simulink model "CELL_MODEL"  (R2017a)
settings: Solver=VariableStepAuto  StartTime=0.0  StopTime=82  RelTol=1e-3
undefined symbols (not defined in the file): C1_LUT, Capacity_LUT, cell_area, cell_Cp_heat, cell_mass, Em_LUT, h_conv, R0_LUT, R1_LUT, SOC_LUT, T_init, Temperature_LUT
settings Model: Creator=Win  LastModifiedBy=Win

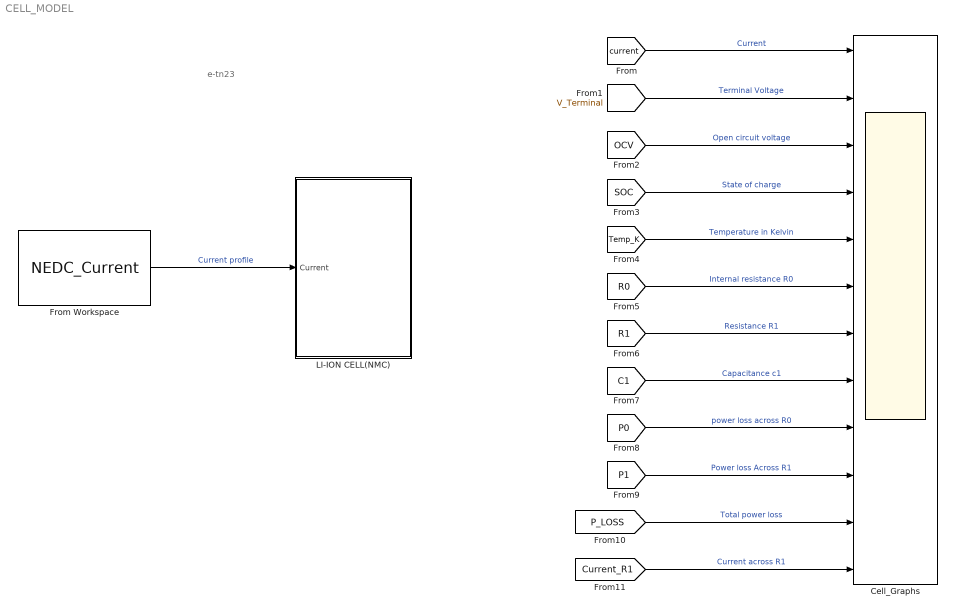
== system CELL_MODEL ==
  note: e-tn23
  Cell_Graphs : Scope  NumInputPorts=12
  From Workspace : FromWorkspace  VariableName=NEDC_Current  SampleTime=0
  LI-ION CELL(NMC) : Subsystem
  wires:
  From Workspace/1 -> LI-ION CELL(NMC)/1(Current)  "Current profile"
  [P_LOSS] -> Cell_Graphs/11  "Total power loss"
  [P1] -> Cell_Graphs/10  "Power loss Across R1"
  [P0] -> Cell_Graphs/9  "power loss across R0"
  [C1] -> Cell_Graphs/8  "Capacitance c1"
  [R1] -> Cell_Graphs/7  "Resistance R1"
  [R0] -> Cell_Graphs/6  "Internal resistance R0"
  [Temp_K] -> Cell_Graphs/5  "Temperature in Kelvin"
  [SOC] -> Cell_Graphs/4  "State of charge"
  [OCV] -> Cell_Graphs/3  "Open circuit voltage"
  [V_Terminal] -> Cell_Graphs/2  "Terminal Voltage"
  [current] -> Cell_Graphs/1  "Current"
  [Current_R1] -> Cell_Graphs/12  "Current across R1"

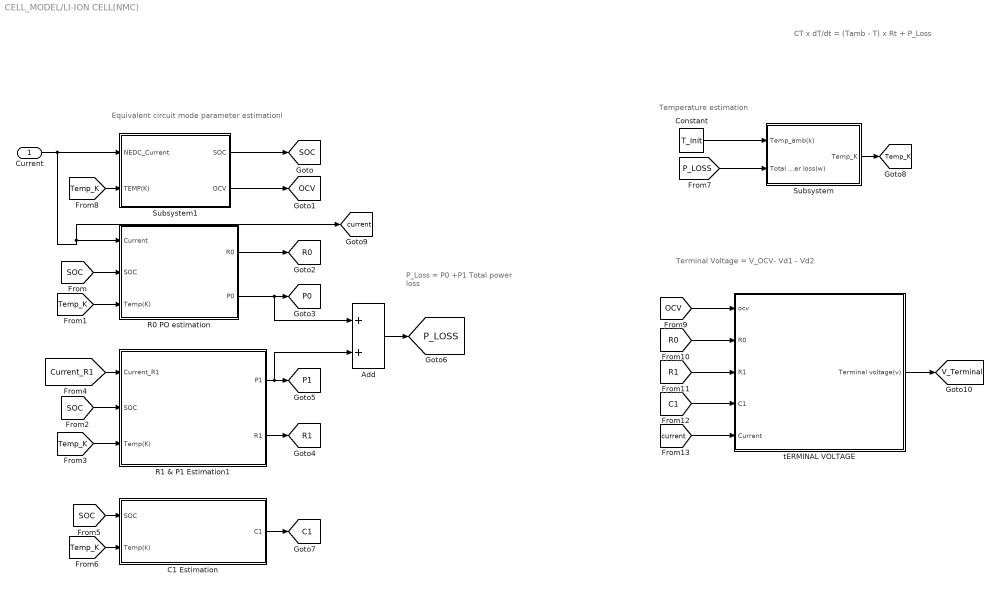
== system CELL_MODEL/LI-ION CELL(NMC) ==
  note: CT x dT/dt = (Tamb - T) x Rt + P_Loss
  note: Terminal Voltage = V_OCV- Vd1 - Vd2
  note: Equivalent circuit mode parameter estimationl
  note: P_Loss = P0 +P1
      | Total power loss
  note: Temperature estimation
  Current : Inport
  Add : Sum
  C1 Estimation : Subsystem
  Constant : Constant  Value=T_init
  R0 PO estimation : Subsystem
  R1 & P1 Estimation1 : Subsystem
  Subsystem : Subsystem
  Subsystem1 : Subsystem
  tERMINAL VOLTAGE : Subsystem
  tag scope: C1=global, OCV=global, P0=global, P1=global, P_LOSS=global, R0=global, R1=global, SOC=global, Temp_K=global, V_Terminal=global, current=global
  wires:
  tERMINAL VOLTAGE/1(Terminal voltage(v)) -> [V_Terminal]
  Add/1 -> [P_LOSS]
  Subsystem1/2(OCV) -> [OCV]
  C1 Estimation/1(C1) -> [C1]
  [R1] -> tERMINAL VOLTAGE/3(R1)
  [current] -> tERMINAL VOLTAGE/5(Current)
  Subsystem1/1(SOC) -> [SOC]
  Constant/1 -> Subsystem/1(Temp_amb(k))
  [OCV] -> tERMINAL VOLTAGE/1(ocv)
  [Temp_K] -> R1 & P1 Estimation1/3(Temp(K))
  [Temp_K] -> Subsystem1/2(TEMP(K))
  [R0] -> tERMINAL VOLTAGE/2(R0)
  [P_LOSS] -> Subsystem/2(Total Power loss(w))
  R0 PO estimation/1(R0) -> [R0]
  [C1] -> tERMINAL VOLTAGE/4(C1)
  [SOC] -> R0 PO estimation/2(SOC)
  [Temp_K] -> C1 Estimation/2(Temp(k))
  R0 PO estimation/2(P0) -> [P0], Add/1
  [SOC] -> R1 & P1 Estimation1/2(SOC)
  Subsystem/1(Temp_K) -> [Temp_K]
  R1 & P1 Estimation1/1(P1) -> Add/2, [P1]
  Current/1 -> [current], R0 PO estimation/1(Current), Subsystem1/1(NEDC_Current)
  [SOC] -> C1 Estimation/1(SOC)
  [Current_R1] -> R1 & P1 Estimation1/1(Current_R1)
  R1 & P1 Estimation1/2(R1) -> [R1]
  [Temp_K] -> R0 PO estimation/3(Temp(K))

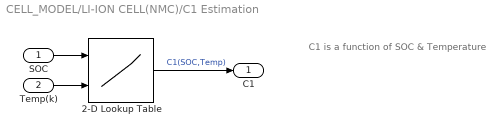
== system CELL_MODEL/LI-ION CELL(NMC)/C1 Estimation ==
  note: C1 is a function of SOC & Temperature
  SOC : Inport
  Temp(k) : Inport  Port=2
  2-D Lookup Table : Lookup_n-D  BreakpointsForDimension1=SOC_LUT  BreakpointsForDimension2=Temperature_LUT  Table=C1_LUT  InternalRulePriority=Speed  RndMeth=Simplest  InputSameDT=on
  C1 : Outport
  wires:
  Temp(k)/1 -> 2-D Lookup Table/2
  SOC/1 -> 2-D Lookup Table/1
  2-D Lookup Table/1 -> C1/1  "C1(SOC,Temp)"

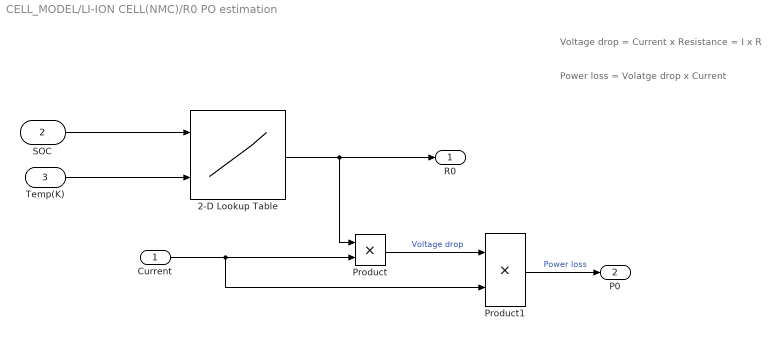
== system CELL_MODEL/LI-ION CELL(NMC)/R0 PO estimation ==
  note: Voltage drop = Current x Resistance = I x R
  note: Power loss = Volatge drop x Current
  Current : Inport
  SOC : Inport  Port=2
  Temp(K) : Inport  Port=3
  2-D Lookup Table : Lookup_n-D  BreakpointsForDimension1=SOC_LUT  BreakpointsForDimension2=Temperature_LUT  Table=R0_LUT  InternalRulePriority=Speed  RndMeth=Simplest  InputSameDT=on
  Product : Product
  Product1 : Product
  R0 : Outport
  P0 : Outport  Port=2
  wires:
  Current/1 -> Product1/2, Product/2
  Product/1 -> Product1/1  "Voltage drop"
  Temp(K)/1 -> 2-D Lookup Table/2
  Product1/1 -> P0/1  "Power loss"
  2-D Lookup Table/1 -> Product/1, R0/1
  SOC/1 -> 2-D Lookup Table/1

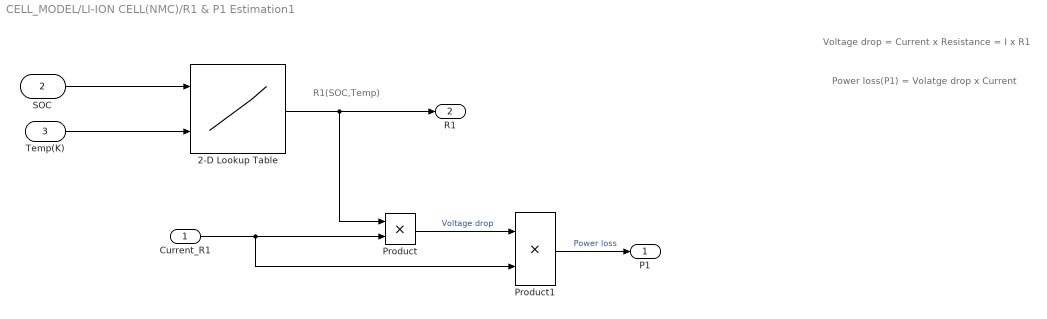
== system CELL_MODEL/LI-ION CELL(NMC)/R1 & P1 Estimation1 ==
  note: R1(SOC,Temp)
  note: Voltage drop = Current x Resistance = I x R1
  note: Power loss(P1) = Volatge drop x Current
  Current_R1 : Inport
  SOC : Inport  Port=2
  Temp(K) : Inport  Port=3
  2-D Lookup Table : Lookup_n-D  BreakpointsForDimension1=SOC_LUT  BreakpointsForDimension2=Temperature_LUT  Table=R1_LUT  InternalRulePriority=Speed  RndMeth=Simplest  InputSameDT=on
  Product : Product
  Product1 : Product
  P1 : Outport
  R1 : Outport  Port=2
  wires:
  Product1/1 -> P1/1  "Power loss"
  Product/1 -> Product1/1  "Voltage drop"
  Current_R1/1 -> Product/2, Product1/2
  2-D Lookup Table/1 -> R1/1, Product/1
  Temp(K)/1 -> 2-D Lookup Table/2
  SOC/1 -> 2-D Lookup Table/1

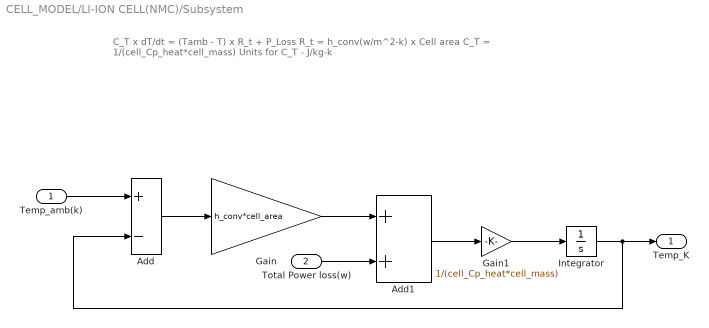
== system CELL_MODEL/LI-ION CELL(NMC)/Subsystem ==
  note: C_T x dT/dt = (Tamb - T) x R_t + P_Loss
      | R_t = h_conv(w/m^2-k) x Cell area
      | C_T = 1/(cell_Cp_heat*cell_mass)
      | Units for C_T - J/kg-k
  Temp_amb(k) : Inport
  Total Power loss(w) : Inport  Port=2
  Add : Sum  Inputs=+-
  Add1 : Sum
  Gain : Gain  Gain=h_conv*cell_area
  Gain1 : Gain  Gain=1/(cell_Cp_heat*cell_mass)
  Integrator : Integrator  InitialCondition=293.15
  Temp_K : Outport
  wires:
  Temp_amb(k)/1 -> Add/1
  Add/1 -> Gain/1
  Gain/1 -> Add1/1
  Total Power loss(w)/1 -> Add1/2
  Add1/1 -> Gain1/1
  Gain1/1 -> Integrator/1
  Integrator/1 -> Add/2, Temp_K/1

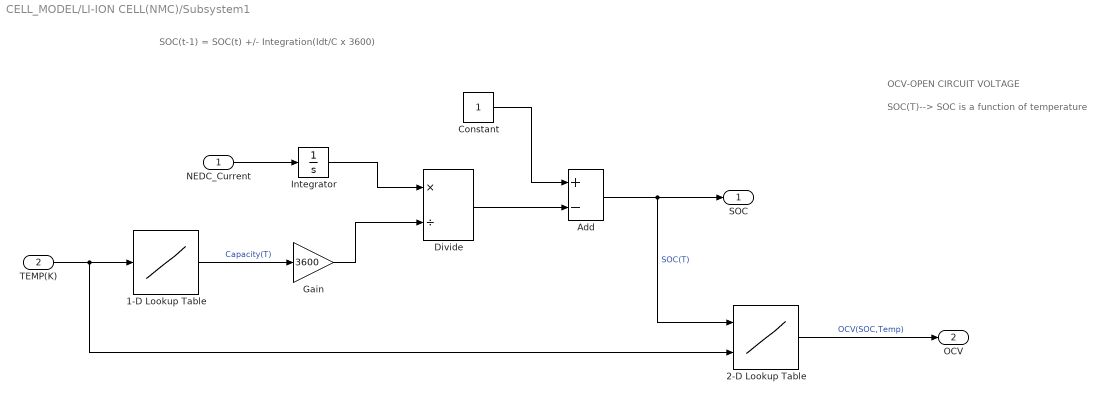
== system CELL_MODEL/LI-ION CELL(NMC)/Subsystem1 ==
  note: OCV-OPEN CIRCUIT VOLTAGE
  note: SOC(T)--> SOC is a function of temperature
  note: SOC(t-1) = SOC(t) +/- Integration(Idt/C x 3600)
  NEDC_Current : Inport
  TEMP(K) : Inport  Port=2
  1-D Lookup Table : Lookup_n-D  NumberOfTableDimensions=1  BreakpointsForDimension1=Temperature_LUT  Table=Capacity_LUT  InternalRulePriority=Speed  RndMeth=Simplest  InputSameDT=on
  2-D Lookup Table : Lookup_n-D  BreakpointsForDimension1=SOC_LUT  BreakpointsForDimension2=Temperature_LUT  Table=Em_LUT  InternalRulePriority=Speed  RndMeth=Simplest  InputSameDT=on
  Add : Sum  Inputs=+-
  Constant : Constant
  Divide : Product  Inputs=*/
  Gain : Gain  Gain=3600
  Integrator : Integrator
  SOC : Outport
  OCV : Outport  Port=2
  wires:
  Divide/1 -> Add/2
  2-D Lookup Table/1 -> OCV/1  "OCV(SOC,Temp)"
  Integrator/1 -> Divide/1
  Add/1 -> 2-D Lookup Table/1, SOC/1  "SOC(T)"
  1-D Lookup Table/1 -> Gain/1  "Capacity(T)"
  Gain/1 -> Divide/2
  TEMP(K)/1 -> 2-D Lookup Table/2, 1-D Lookup Table/1
  NEDC_Current/1 -> Integrator/1
  Constant/1 -> Add/1

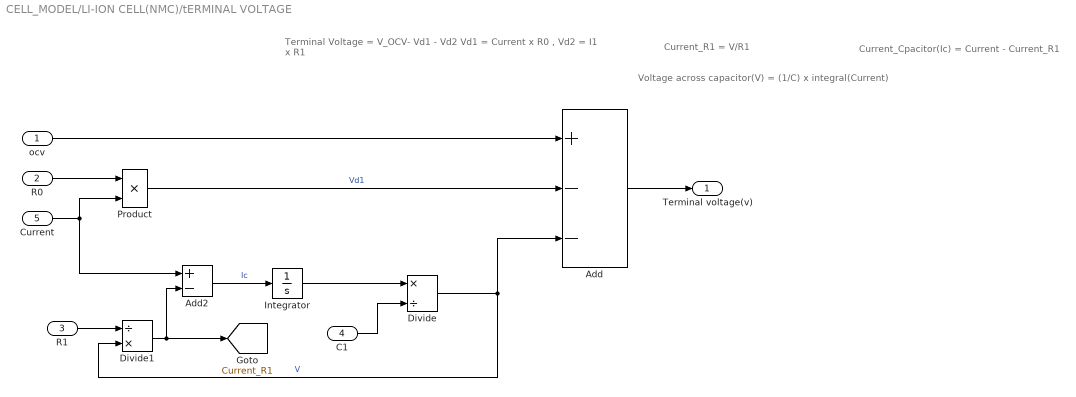
== system CELL_MODEL/LI-ION CELL(NMC)/tERMINAL VOLTAGE ==
  note: Current_Cpacitor(Ic) = Current - Current_R1
  note: Voltage across capacitor(V) = (1/C) x integral(Current)
  note: Current_R1 = V/R1
  note: Terminal Voltage = V_OCV- Vd1 - Vd2
      | Vd1 = Current x R0 , Vd2 = I1 x R1
  ocv : Inport
  R0 : Inport  Port=2
  R1 : Inport  Port=3
  C1 : Inport  Port=4
  Current : Inport  Port=5
  Add : Sum  Inputs=+--
  Add2 : Sum  Inputs=+-
  Divide : Product  Inputs=*/
  Divide1 : Product  Inputs=/*
  Integrator : Integrator
  Product : Product
  Terminal voltage(v) : Outport
  tag scope: Current_R1=global
  wires:
  Add/1 -> Terminal voltage(v)/1
  ocv/1 -> Add/1
  R0/1 -> Product/1
  Current/1 -> Add2/1, Product/2
  Product/1 -> Add/2  "Vd1"
  C1/1 -> Divide/2
  Divide/1 -> Divide1/2, Add/3  "V"
  R1/1 -> Divide1/1
  Divide1/1 -> [Current_R1], Add2/2
  Add2/1 -> Integrator/1  "Ic"
  Integrator/1 -> Divide/1
